simulink model "zsim"  (R2020b)
settings: Solver=ode45  StartTime=0.0  StopTime=20  RelTol=1e-5  EnableMultiTasking=on
settings Model: ExtModeTrigMode=oneshot  ExtModeArmWhenConnect=off  Creator=ljk  LastModifiedBy=zhang lei
settings SolverCC: AlgebraicLoopSolver=LineSearch
settings DataIOCC: SaveFormat=Array  SignalLoggingSaveFormat=ModelDataLogs  ReturnWorkspaceOutputs=off  SignalLoggingName=sigsOut
settings OptimizationCC: BooleanDataType=off  ExpressionDepthLimit=2147483647  InitFltsAndDblsToZero=on  LifeSpan=inf
settings DebuggingCC: SaveWithParameterizedLinksMsg=none  UnderspecifiedInitializationDetection=Classic  MergeDetectMultiDrivingBlocksExec=none  SignalResolutionControl=TryResolveAllWithWarning  MultiTaskDSMMsg=warning  MultiTaskCondExecSysMsg=none  FcnCallInpInsideContextMsg=warning  StateNameClashWarn=warning  SFUnexpectedBacktrackingDiag=warning  SFNoUnconditionalDefaultTransitionDiag=warning  SFExecutionAtInitializationDiag=none  ArithmeticOperatorsInVariantConditions=warning
settings HardwareCC: ProdBitPerPointer=32  ProdBitPerSizeT=32  ProdBitPerPtrDiffT=32  ProdLargestAtomicFloat=None  ProdIntDivRoundTo=Undefined  ProdEndianess=Unspecified  ProdWordSize=32  ProdHWDeviceType=32-bit Generic  TargetUnknown=on
settings ModelReferenceCC: PropagateSignalLabelsOutOfModel=off
settings SFSimCC: SimUseLocalCustomCode=off  CustomCodeUndefinedFunction=UseInterfaceOnly
settings RTWCC: RTWUseLocalCustomCode=off
settings CodeAppCC: StateflowObjectComments=on
settings GRTTargetCC: TargetFcnLib=ansi_tfl_tmw.mat  TargetLangStandard=C89/C90 (ANSI)  CombineOutputUpdateFcns=off  GRTInterface=on
settings ConfigComp: CovMetricSettings=dw  CovSaveCumulativeToWorkspaceVar=on  CovSaveSingleToWorkspaceVar=on  CovExternalEMLEnable=off  CovSFcnEnable=off

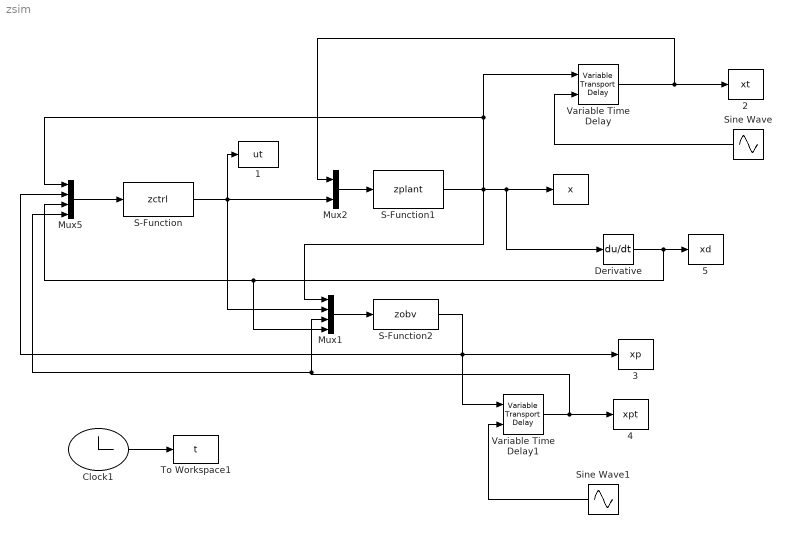
== system zsim ==
  "  " : ToWorkspace  VariableName=x  SampleTime=-1
  "  1" : ToWorkspace  VariableName=ut  SampleTime=-1
  "  2" : ToWorkspace  VariableName=xt  SampleTime=-1
  "  3" : ToWorkspace  VariableName=xp  SampleTime=-1
  "  4" : ToWorkspace  VariableName=xpt  SampleTime=-1
  "  5" : ToWorkspace  VariableName=xd  SampleTime=-1
  Clock1 : Clock
  Derivative : Derivative
  Mux1 : Mux
  Mux2 : Mux  Inputs=2
  Mux5 : Mux
  "S-Function " : S-Function  FunctionName=zctrl  SFunctionDeploymentMode=off  EnableBusSupport=off
  S-Function1 : S-Function  FunctionName=zplant  SFunctionDeploymentMode=off  EnableBusSupport=off
  S-Function2 : S-Function  FunctionName=zobv  SFunctionDeploymentMode=off  EnableBusSupport=off
  Sine Wave : Sin  Amplitude=0.5  Bias=1  SampleTime=0
  Sine Wave1 : Sin  Amplitude=0.5  Bias=1  SampleTime=0
  To Workspace1 : ToWorkspace  VariableName=t  SampleTime=-1
  Variable Time Delay : VariableTransportDelay  MaximumDelay=10  ZeroDelay=on
  Variable Time Delay1 : VariableTransportDelay  MaximumDelay=10  ZeroDelay=on
  wires:
  S-Function2/1 -> Variable Time Delay1/1, "  3"/1, Mux5/2
  "S-Function "/1 -> "  1"/1, Mux2/2, Mux1/2
  Clock1/1 -> To Workspace1/1
  Mux1/1 -> S-Function2/1
  S-Function1/1 -> Mux1/1, Variable Time Delay/1, Mux5/1, Derivative/1, "  "/1
  Mux2/1 -> S-Function1/1
  Variable Time Delay/1 -> "  2"/1, Mux2/1
  Variable Time Delay1/1 -> Mux5/4, Mux1/3, "  4"/1
  Mux5/1 -> "S-Function "/1
  Derivative/1 -> Mux1/4, Mux5/3, "  5"/1
  Sine Wave/1 -> Variable Time Delay/2
  Sine Wave1/1 -> Variable Time Delay1/2
